simulink model "untitled"  (R2021a)
settings: Solver=VariableStepAuto  StartTime=0.0  StopTime=10.0  RelTol=1e-3
settings Model: Creator=User  LastModifiedBy=User

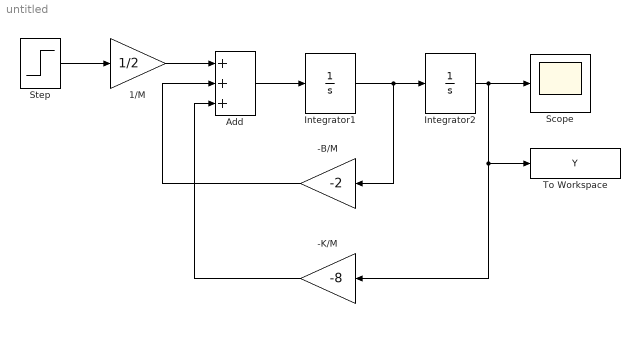
== system untitled ==
  -B/M : Gain  Gain=-2
  -K/M : Gain  Gain=-8
  1/M : Gain  Gain=1/2
  Add : Sum  Inputs=+++
  Integrator1 : Integrator
  Integrator2 : Integrator
  Scope : Scope
  Step : Step  SampleTime=0
  To Workspace : ToWorkspace  VariableName=Y  SaveFormat=Timeseries  SampleTime=-1
  wires:
  Step/1 -> 1/M/1
  1/M/1 -> Add/1
  Add/1 -> Integrator1/1
  Integrator1/1 -> -B/M/1, Integrator2/1
  Integrator2/1 -> To Workspace/1, -K/M/1, Scope/1
  -B/M/1 -> Add/2
  -K/M/1 -> Add/3
